simulink model "Simulink_Deliverable1_2_"  (R2025a)
settings: Solver=FixedStepAuto  StartTime=0.0  StopTime=10.0  FixedStep=1e-3  RelTol=1e-3  EnableMultiTasking=on
undefined symbols (not defined in the file): A0, A1, A2, A3, A4, D0, D1, D10, D11, D12, D13, D2, D3, D4, D5, D6, D7, D8, D9, PTA0, PTA1, PTA2, PTB10, PTB11, PTB2, PTB23, PTB3, PTB9, PTC11, PTC16, PTC17, PTC2, PTC3, PTC4, PTD0, PTD1, PTD2, PTD3
libraries: frdmk64flib x19
settings Model: ExtModeTrigDuration=5  Creator=shaun  LastModifiedBy=anila
settings OptimizationCC: DefaultParameterBehavior=Inlined  EnhancedBackFolding=on  PassReuseOutputArgsAs=Individual arguments  ZeroExternalMemoryAtStartup=off  ZeroInternalMemoryAtStartup=off  MaxStackSize=64  OptimizeBlockOrder=speed  DifferentSizesBufferReuse=on  OptimizationCustomize=off  EfficientTunableParamExpr=on
settings DebuggingCC: ParameterTunabilityLossMsg=error
settings HardwareCC: ProdBitPerPointer=32.0  ProdBitPerSizeT=32.0  ProdBitPerPtrDiffT=32.0  ProdLargestAtomicInteger=Long  ProdLargestAtomicFloat=Double  ProdWordSize=32.0  ProdHWDeviceType=ARM Compatible->ARM Cortex
settings SFSimCC: MATLABDynamicMemAlloc=off
settings RTWCC: SystemTargetFile=ert.tlc  HardwareBoard=NXP FRDM-K64F  TLCOptions="-aInlineSetEventsForThisBaseRateFcn=TLC_FALSE -aSuppressMultiTaskScheduler=TLC_FALSE  -aRateBasedStepFcn=0"  TemplateMakefile=ert_default_tmf  Toolchain=GNU Tools for ARM Embedded Processors  Description=Embedded Coder
settings CodeAppCC: ForceParamTrailComments=on  IgnoreCustomStorageClasses=off  OperatorAnnotations=on  SimulinkDataObjDesc=on  SFDataObjDesc=on  InsertBlockDesc=on
settings ERTTargetCC: ExtModeTransport=4.0  ExtModeStaticAlloc=off  ExtModeMexFile=sendToCommService  ExtModeIntrfLevel=Level1

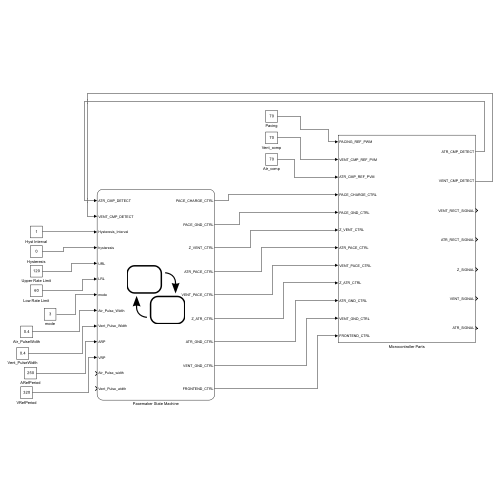
[thumbnail: Simulink's stored preview of the top-level diagram]
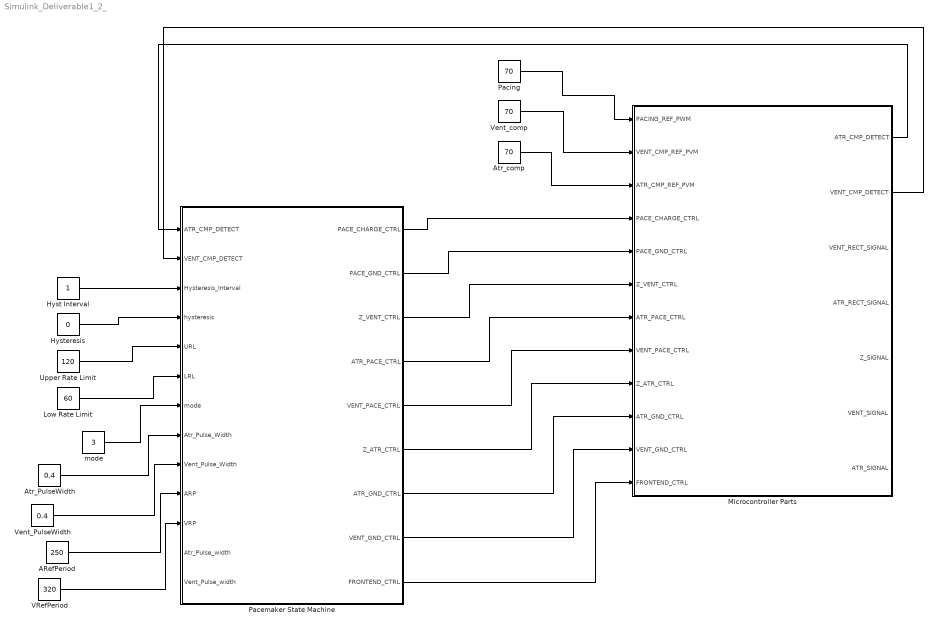
== system Simulink_Deliverable1_2_ ==
  ARefPeriod : Constant  Value=250
  Atr_PulseWidth : Constant  Value=0.4
  Atr_comp : Constant  Value=70
  Hyst Interval : Constant
  Hysteresis : Constant  Value=0
  Low Rate Limit : Constant  Value=60
  Microcontroller Parts : Subsystem
  Pacemaker State Machine : Stateflow chart  TreatAsAtomicUnit=on
  Pacing : Constant  Value=70
  Upper Rate Limit : Constant  Value=120
  VRefPeriod : Constant  Value=320
  Vent_PulseWidth : Constant  Value=0.4
  Vent_comp : Constant  Value=70
  mode : Constant  Value=3
  wires:
  Pacemaker State Machine/1(PACE_CHARGE_CTRL) -> Microcontroller Parts/4(PACE_CHARGE_CTRL)
  Pacemaker State Machine/2(PACE_GND_CTRL) -> Microcontroller Parts/5(PACE_GND_CTRL)
  Pacemaker State Machine/3(Z_VENT_CTRL) -> Microcontroller Parts/6(Z_VENT_CTRL)
  Pacemaker State Machine/4(ATR_PACE_CTRL) -> Microcontroller Parts/7(ATR_PACE_CTRL)
  Pacemaker State Machine/5(VENT_PACE_CTRL) -> Microcontroller Parts/8(VENT_PACE_CTRL)
  Pacemaker State Machine/6(Z_ATR_CTRL) -> Microcontroller Parts/9(Z_ATR_CTRL)
  Pacemaker State Machine/7(ATR_GND_CTRL) -> Microcontroller Parts/10(ATR_GND_CTRL)
  Pacemaker State Machine/8(VENT_GND_CTRL) -> Microcontroller Parts/11(VENT_GND_CTRL)
  Pacemaker State Machine/9(FRONTEND_CTRL) -> Microcontroller Parts/12(FRONTEND_CTRL)
  Pacing/1 -> Microcontroller Parts/1(PACING_REF_PWM)
  Vent_comp/1 -> Microcontroller Parts/2(VENT_CMP_REF_PVM)
  Atr_comp/1 -> Microcontroller Parts/3(ATR_CMP_REF_PVM)
  Microcontroller Parts/2(VENT_CMP_DETECT) -> Pacemaker State Machine/2(VENT_CMP_DETECT)
  Hyst Interval/1 -> Pacemaker State Machine/3(Hysteresis_Interval)
  Hysteresis/1 -> Pacemaker State Machine/4(hysteresis)
  Upper Rate Limit/1 -> Pacemaker State Machine/5(URL)
  Low Rate Limit/1 -> Pacemaker State Machine/6(LRL)
  mode/1 -> Pacemaker State Machine/7(mode)
  Atr_PulseWidth/1 -> Pacemaker State Machine/8(Atr_Pulse_Width)
  Vent_PulseWidth/1 -> Pacemaker State Machine/9(Vent_Pulse_Width)
  ARefPeriod/1 -> Pacemaker State Machine/10(ARP)
  VRefPeriod/1 -> Pacemaker State Machine/11(VRP)
  Microcontroller Parts/1(ATR_CMP_DETECT) -> Pacemaker State Machine/1(ATR_CMP_DETECT)

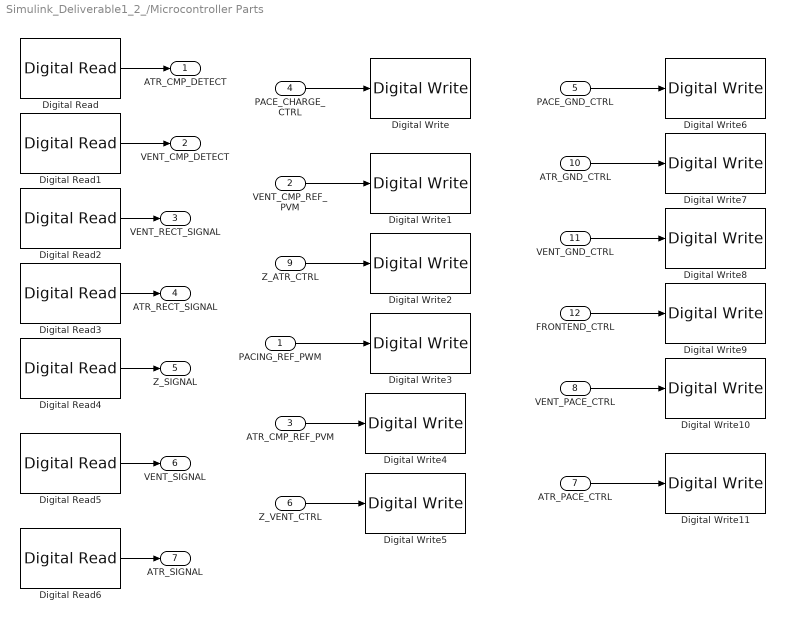
== system Simulink_Deliverable1_2_/Microcontroller Parts ==
  PACING_REF_PWM : Inport
  VENT_CMP_REF_PVM : Inport  Port=2
  ATR_CMP_REF_PVM : Inport  Port=3
  PACE_CHARGE_CTRL : Inport  Port=4
  PACE_GND_CTRL : Inport  Port=5
  Z_VENT_CTRL : Inport  Port=6
  ATR_PACE_CTRL : Inport  Port=7
  VENT_PACE_CTRL : Inport  Port=8
  Z_ATR_CTRL : Inport  Port=9
  ATR_GND_CTRL : Inport  Port=10
  VENT_GND_CTRL : Inport  Port=11
  FRONTEND_CTRL : Inport  Port=12
  Digital Read : frdmk64flib/Digital Read  Whichpin=PTC16 (D0)  SampleTime=-1
  Digital Read1 : frdmk64flib/Digital Read  Whichpin=PTC17 (D1)  SampleTime=-1
  Digital Read2 : frdmk64flib/Digital Read  Whichpin=PTC11 (A4)  SampleTime=-1
  Digital Read3 : frdmk64flib/Digital Read  Whichpin=PTB11 (A3)  SampleTime=-1
  Digital Read4 : frdmk64flib/Digital Read  Whichpin=PTB10 (A2)  SampleTime=-1
  Digital Read5 : frdmk64flib/Digital Read  Whichpin=PTB3 (A1)  SampleTime=-1
  Digital Read6 : frdmk64flib/Digital Read  Whichpin=PTB2 (A0)  SampleTime=-1
  Digital Write : frdmk64flib/Digital Write  Whichpin=PTB9 (D2)
  Digital Write1 : frdmk64flib/Digital Write  Whichpin=PTA1 (D3)
  Digital Write10 : frdmk64flib/Digital Write  Whichpin=PTA0 (D8)
  Digital Write11 : frdmk64flib/Digital Write  Whichpin=PTC4 (D9)
  Digital Write2 : frdmk64flib/Digital Write  Whichpin=PTB23 (D4)
  Digital Write3 : frdmk64flib/Digital Write  Whichpin=PTA2 (D5)
  Digital Write4 : frdmk64flib/Digital Write  Whichpin=PTC2 (D6)
  Digital Write5 : frdmk64flib/Digital Write  Whichpin=PTC3 (D7)
  Digital Write6 : frdmk64flib/Digital Write  Whichpin=PTD0 (D10)
  Digital Write7 : frdmk64flib/Digital Write  Whichpin=PTD2 (D11)
  Digital Write8 : frdmk64flib/Digital Write  Whichpin=PTD3 (D12)
  Digital Write9 : frdmk64flib/Digital Write  Whichpin=PTD1 (D13)
  ATR_CMP_DETECT : Outport
  VENT_CMP_DETECT : Outport  Port=2
  VENT_RECT_SIGNAL : Outport  Port=3
  ATR_RECT_SIGNAL : Outport  Port=4
  Z_SIGNAL : Outport  Port=5
  VENT_SIGNAL : Outport  Port=6
  ATR_SIGNAL : Outport  Port=7
  wires:
  Digital Read/1 -> ATR_CMP_DETECT/1
  Digital Read1/1 -> VENT_CMP_DETECT/1
  Digital Read2/1 -> VENT_RECT_SIGNAL/1
  Digital Read3/1 -> ATR_RECT_SIGNAL/1
  Digital Read4/1 -> Z_SIGNAL/1
  Digital Read5/1 -> VENT_SIGNAL/1
  Digital Read6/1 -> ATR_SIGNAL/1
  PACE_CHARGE_CTRL/1 -> Digital Write/1
  VENT_CMP_REF_PVM/1 -> Digital Write1/1
  Z_ATR_CTRL/1 -> Digital Write2/1
  PACING_REF_PWM/1 -> Digital Write3/1
  ATR_CMP_REF_PVM/1 -> Digital Write4/1
  Z_VENT_CTRL/1 -> Digital Write5/1
  PACE_GND_CTRL/1 -> Digital Write6/1
  ATR_GND_CTRL/1 -> Digital Write7/1
  VENT_GND_CTRL/1 -> Digital Write8/1
  FRONTEND_CTRL/1 -> Digital Write9/1
  VENT_PACE_CTRL/1 -> Digital Write10/1
  ATR_PACE_CTRL/1 -> Digital Write11/1

== stateflow chart Simulink_Deliverable1_2_/Pacemaker State Machine ==
  state VII
    state ChargeSense
      entry:
      PACE_GND_CTRL=true;
      VENT_GND_CTRL=true;
      FRONTEND_CTRL=true;
      PACE_CHARGE_CTRL=true;
      VENT_PACE_CTRL=false;
      Z_VENT_CTRL=true;
      % switch off all
      Z_ATR_CTRL = false;
      ATR_PACE_CTRL = false;
      ATR_GND_CTRL = false;
    state HYSTERESIS
      entry:
      PACE_CHARGE_CTRL = true;
      FRONTEND_CTRL = true;
      % ventricall pace control charged up (on)
      Z_VENT_CTRL = false;
      VENT_GND_CTRL = false;
      PACE_GND_CTRL = true;
      VENT_PACE_CTRL = true;
    state VPACE
      entry:
      PACE_CHARGE_CTRL = false;
      FRONTEND_CTRL = false;
      % ventrical pace control not charged (off)
      Z_VENT_CTRL = false;
      VENT_GND_CTRL = false;
      VENT_PACE_CTRL = true;
    (default) -> ChargeSense
    VPACE -> ChargeSense : [after(LRL-Vent_Pulse_Width,msec)]
    HYSTERESIS -> VPACE [order 1] : [after(LRL+Hysteresis_Interval,msec)]
    ChargeSense -> VPACE [order 1] : [after(LRL-Vent_Pulse_Width,msec) && after(URL-Vent_Pulse_Width,msec)]
    ChargeSense -> HYSTERESIS [order 3] : [hysteresis == true && VENT_CMP_DETECT == true && after(VRP,msec)]
    HYSTERESIS -> HYSTERESIS [order 2] : [hysteresis == true && VENT_CMP_DETECT == true && after(VRP,msec)]
    ChargeSense -> ChargeSense [order 2] : [hysteresis == false && VENT_CMP_DETECT == true && after(VRP,msec)]
  state AOO
    state ChargingDischarging
      entry:
      PACE_CHARGE_CTRL = true;    % turn on charging of pacing capacitor
      FRONTEND_CTRL = false;    % disable sensing
      ATR_PACE_CTRL = false;    % turn off pacing for charge stage
      VENT_PACE_CTRL = false;    % no ventricular pacing
      PACE_GND_CTRL = true;     % keep pacing cap circuit closed
      ATR_GND_CTRL = true;        % keep atrium grounded
      VENT_GND_CTRL = false;    % no grounding for vent side
      % disable impedance measurement (both atr and vent)
      Z_ATR_CTRL = false;
      Z_VENT_CTRL = false;
    state APacing
      entry:
      PACE_CHARGE_CTRL = false;    % stop charging pacing capacitor
      ATR_PACE_CTRL = true;    % enable the atrial pacing output
      VENT_PACE_CTRL = false;    % no ventricular pacing
      ATR_GND_CTRL = false;    % no atrial ground during pacing output
      PACE_GND_CTRL = true;    % ground to complete pacing circuit
      VENT_GND_CTRL = false;    % no grounding for vent side
      % disable impedance measurement (both atr and vent)
      Z_ATR_CTRL = false;
      Z_VENT_CTRL = false;
    (default) -> AOO.ChargingDischarging
    AOO.ChargingDischarging -> APacing : [after(LRL-Atr_Pulse_Width,msec) && after(URL - Atr_Pulse_width,msec)]
    APacing -> AOO.ChargingDischarging : [after(Atr_Pulse_Width, msec)]
  state Choose_mode
  state VOO
    state ChargingDischarging
      entry:
      PACE_CHARGE_CTRL = true;    % enable charging pacing capacitor
      FRONTEND_CTRL = false;    % disable sensing
      ATR_PACE_CTRL = false;    % no pacing when charging pacing capacitor
      VENT_PACE_CTRL = false;    % no ventricular pacing
      PACE_GND_CTRL = true;    % enable ground for pace cap
      ATR_GND_CTRL = false;    % keep atrial ground enabled
      VENT_GND_CTRL = true;    % no ventricular ground
      % disable impedance measurement (both atr and vent)
      Z_VENT_CTRL = false;
      Z_ATR_CTRL = false;
    state VPacing
      entry:
      PACE_CHARGE_CTRL = false;    % stop charging pacing capacitor
      ATR_PACE_CTRL = false;    % enable atrial pacing output
      VENT_PACE_CTRL = true;    % no ventricular pacing
      PACE_GND_CTRL = true;    % close pacing capacitor, discharge
      ATR_GND_CTRL = false;    % turn off atrial grounding for pacing
      VENT_GND_CTRL = false;  % no ventricular ground
      % disable impedance measurement (both atr and vent)
      Z_VENT_CTRL = false;
      Z_ATR_CTRL = false;
    (default) -> VOO.ChargingDischarging
    VOO.ChargingDischarging -> VPacing : [after(LRL-Vent_Pulse_Width,msec) && after(URL - Vent_Pulse_width,msec)]
    VPacing -> VOO.ChargingDischarging : [after(Vent_Pulse_Width, msec)]
  state AAI
    state AtrialPacing
      entry:
      %Pacing stage
      FRONTEND_CTRL = false;
      %Discharge pacing capacitor
      PACE_CHARGE_CTRL = false;
      VENT_PACE_CTRL = false;
      ATR_PACE_CTRL = true;
      %Ground controlling
      PACE_GND_CTRL = true;
      VENT_GND_CTRL = false;
      ATR_GND_CTRL = false;
      %Lead impedance measurement
      Z_VENT_CTRL = false;
      Z_ATR_CTRL = false;
    state Hysteresis
      entry:
      %Sensing stage
      FRONTEND_CTRL = true;
      %Charge pacing capacitor
      PACE_CHARGE_CTRL = true;
      VENT_PACE_CTRL = false;
      ATR_PACE_CTRL = false;
      %Ground controlling
      PACE_GND_CTRL = true;
      VENT_GND_CTRL = false;
      ATR_GND_CTRL = true;
      %Lead impedance measurement
      Z_VENT_CTRL = false;
      Z_ATR_CTRL = false;
    state AtrialSensing
      %Sensing stage
      FRONTEND_CTRL = true;
      %Charging capacitor
      PACE_CHARGE_CTRL = true;
      VENT_PACE_CTRL = false;
      ATR_PACE_CTRL = false;
      %Ground controlling
      PACE_GND_CTRL = true;
      VENT_GND_CTRL = false;
      ATR_GND_CTRL = true;
      %Lead impedance measurement
      Z_VENT_CTRL = false;
      Z_ATR_CTRL = false;
    (default) -> AtrialSensing
    Hysteresis -> Hysteresis [order 2] : [hysteresis == true && ATR_CMP_DETECT == true && after(ARP, msec)]
    AtrialSensing -> AtrialPacing [order 1] : [after(LRL-Atr_Pulse_Width,msec) && after(URL-Atr_Pulse_Width,msec)]
    Hysteresis -> AtrialPacing [order 1] : [after(LRL+Hysteresis_Interval,msec)]
    AtrialPacing -> AtrialSensing : [after(Atr_Pulse_Width,msec)]
    AtrialSensing -> AtrialSensing [order 2] : [hysteresis == false && ATR_CMP_DETECT == true && after(ARP, msec)]
    AtrialSensing -> Hysteresis [order 3] : [hysteresis == true && ATR_CMP_DETECT == true && after(ARP, msec)]
  Choose_mode -> VII [order 2] : [mode == 3]
  Choose_mode -> AOO [order 3] : [mode ==0]
  (default) -> Choose_mode
  Choose_mode -> AAI [order 1] : [mode == 2]
  Choose_mode -> VOO [order 4] : [mode ==1]
  data: PACE_CHARGE_CTRL output; PACE_GND_CTRL output; Z_VENT_CTRL output; ATR_PACE_CTRL output; VENT_PACE_CTRL output; Z_ATR_CTRL output; ATR_GND_CTRL output; VENT_GND_CTRL output; ATR_CMP_DETECT input; VENT_CMP_DETECT input; Hysteresis_Interval input; hysteresis input; URL input; LRL input; mode input; Atr_Pulse_Width input; Vent_Pulse_Width input; ARP input; VRP input; FRONTEND_CTRL output; Atr_Pulse_width input; Vent_Pulse_width input
